simulink model "task9_8"  (R2021a)
settings: Solver=VariableStepAuto  StartTime=0.0  StopTime=10.0  RelTol=1e-3
settings Model: Creator=reemb  LastModifiedBy=reemb

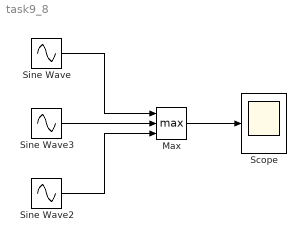
== system task9_8 ==
  Max : MinMax  Function=max  Inputs=3
  Scope : Scope
  Sine Wave : Sin  SampleTime=0
  Sine Wave2 : Sin  Phase=(2*pi/3)  SampleTime=0
  Sine Wave3 : Sin  Phase=pi/3  SampleTime=0
  wires:
  Max/1 -> Scope/1
  Sine Wave/1 -> Max/1
  Sine Wave3/1 -> Max/2
  Sine Wave2/1 -> Max/3
